simulink model "type_check"  (R2017b)
settings: Solver=VariableStepAuto  StartTime=0.0  StopTime=10.0  RelTol=1e-3
settings Model: Creator=cyarp  LastModifiedBy=cyarp
settings OptimizationCC: BlockReduction=off  ConditionallyExecuteInputs=off  DefaultParameterBehavior=Inlined
settings DebuggingCC: AlgebraicLoopMsg=error
settings HardwareCC: ProdBitPerPointer=32  ProdBitPerSizeT=32  ProdBitPerPtrDiffT=32  ProdLargestAtomicFloat=None  ProdIntDivRoundTo=Undefined  ProdEndianess=Unspecified  ProdWordSize=32  ProdHWDeviceType=ASIC/FPGA->ASIC/FPGA  TargetBitPerLong=64  TargetBitPerPointer=64  TargetBitPerSizeT=64  TargetBitPerPtrDiffT=64  TargetLongLongMode=on  TargetIntDivRoundTo=Zero  TargetEndianess=LittleEndian  TargetWordSize=64  TargetHWDeviceType=Custom Processor->MATLAB Host Computer  ProdEqTarget=off

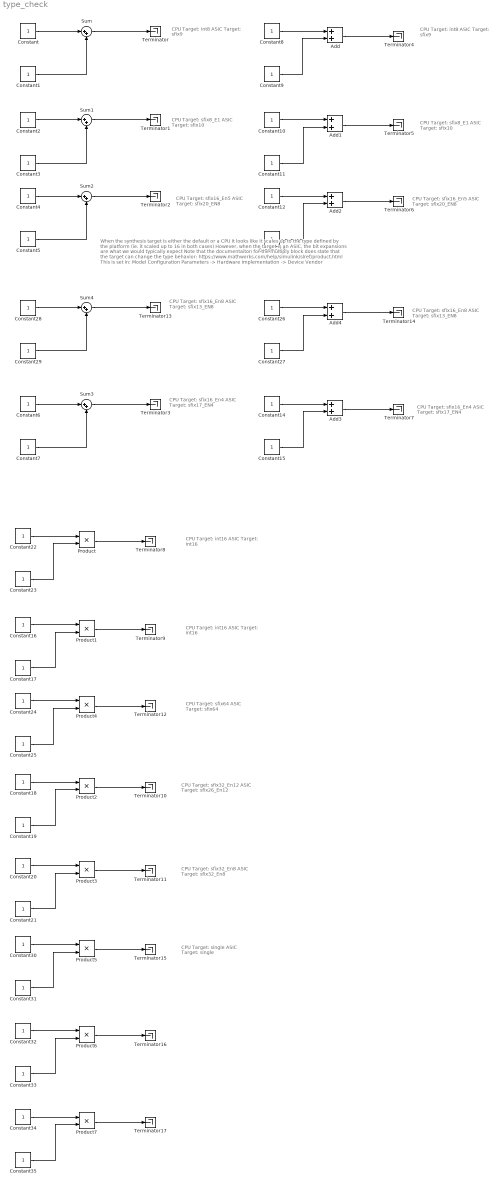
== system type_check ==
  note: CPU Target: sfix16_En5
      | ASIC Target: sfix20_EN8
  note: When the synthesis target is either the default or a CPU
      |
      | It looks like it scales up to the type
      | defined by the platform (ie. it scaled up to 16 in both cases)
      |
      | However, when the target is an ASIC, the bit expansions are what we would typically expect
      |
      | Note that the documentaiton for the multiply block does state that the target can change the type behavior:
      | https://www.mathworks.com/help/simulink/slref/product.html
      |
      | This is set in: Model Configuration Parameters -> Hardware Implementation -> Device Vendor
  note: CPU Target: sfix16_En5
      | ASIC Target: sfix20_EN8
  note: CPU Target: sfix16_En8
      | ASIC Target: sfix13_EN8
  note: CPU Target: sfix16_En8
      | ASIC Target: sfix13_EN8
  note: CPU Target: sfix16_En4
      | ASIC Target: sfix17_EN4
  note: CPU Target: sfix16_En4
      | ASIC Target: sfix17_EN4
  note: CPU Target: int8
      | ASIC Target: sfix9
  note: CPU Target: int8
      | ASIC Target: sfix9
  note: CPU Target: sfix8_E1
      | ASIC Target: sfix10
  note: CPU Target: sfix8_E1
      | ASIC Target: sfix10
  note: CPU Target:  int16
      | ASIC Target: int16
  note: CPU Target:  int16
      | ASIC Target: int16
  note: CPU Target:  sfix64
      | ASIC Target: sfix64
  note: CPU Target:  sfix32_En12
      | ASIC Target: sfix26_En12
  note: CPU Target:  sfix32_En8
      | ASIC Target: sfix32_En8
  note: CPU Target:  single
      | ASIC Target: single
  Add{,1..4} (5 alike) : Sum
  Constant{,1..2,8..10,16,22..23} (9 alike) : Constant  OutDataTypeStr=int8
  Constant11 : Constant  OutDataTypeStr=uint8
  Constant12 : Constant  OutDataTypeStr=fixdt(1,15,4)
  Constant{5,13,19,27,29} (5 alike) : Constant  OutDataTypeStr=fixdt(1,10,8)
  Constant{6..7,14..15,18,20..21,32} (8 alike) : Constant  OutDataTypeStr=fixdt(1,16,4)
  Constant17 : Constant  OutDataTypeStr=uint8
  Constant24 : Constant  OutDataTypeStr=int32
  Constant25 : Constant  OutDataTypeStr=int32
  Constant26 : Constant  OutDataTypeStr=fixdt(1,8,4)
  Constant28 : Constant  OutDataTypeStr=fixdt(1,8,4)
  Constant3 : Constant  OutDataTypeStr=uint8
  Constant30 : Constant  OutDataTypeStr=single
  Constant31 : Constant  OutDataTypeStr=single
  Constant33 : Constant  OutDataTypeStr=double
  Constant34 : Constant  OutDataTypeStr=single
  Constant35 : Constant  OutDataTypeStr=double
  Constant4 : Constant  OutDataTypeStr=fixdt(1,15,4)
  Product{,1..7} (8 alike) : Product
  Sum{,1..4} (5 alike) : Sum  Inputs=|++
  Terminator{,1..17} (18 alike) : Terminator
  wires:
  Constant/1 -> Sum/1
  Constant1/1 -> Sum/2
  Sum/1 -> Terminator/1
  Constant3/1 -> Sum1/2
  Sum1/1 -> Terminator1/1
  Constant2/1 -> Sum1/1
  Sum2/1 -> Terminator2/1
  Constant5/1 -> Sum2/2
  Constant4/1 -> Sum2/1
  Constant7/1 -> Sum3/2
  Constant6/1 -> Sum3/1
  Sum3/1 -> Terminator3/1
  Add/1 -> Terminator4/1
  Constant8/1 -> Add/1
  Constant9/1 -> Add/2
  Constant10/1 -> Add1/1
  Constant11/1 -> Add1/2
  Add1/1 -> Terminator5/1
  Constant12/1 -> Add2/1
  Constant13/1 -> Add2/2
  Add2/1 -> Terminator6/1
  Constant14/1 -> Add3/1
  Constant15/1 -> Add3/2
  Add3/1 -> Terminator7/1
  Constant16/1 -> Product1/1
  Constant18/1 -> Product2/1
  Constant21/1 -> Product3/2
  Constant19/1 -> Product2/2
  Constant20/1 -> Product3/1
  Constant22/1 -> Product/1
  Product1/1 -> Terminator9/1
  Product/1 -> Terminator8/1
  Constant17/1 -> Product1/2
  Product2/1 -> Terminator10/1
  Product3/1 -> Terminator11/1
  Constant23/1 -> Product/2
  Product4/1 -> Terminator12/1
  Constant25/1 -> Product4/2
  Constant24/1 -> Product4/1
  Constant26/1 -> Add4/1
  Constant27/1 -> Add4/2
  Sum4/1 -> Terminator13/1
  Constant29/1 -> Sum4/2
  Constant28/1 -> Sum4/1
  Add4/1 -> Terminator14/1
  Product5/1 -> Terminator15/1
  Constant31/1 -> Product5/2
  Constant30/1 -> Product5/1
  Constant32/1 -> Product6/1
  Product6/1 -> Terminator16/1
  Constant33/1 -> Product6/2
  Product7/1 -> Terminator17/1
  Constant34/1 -> Product7/1
  Constant35/1 -> Product7/2
